simulink model "sensorless_pll_learning"  (R2025b)
settings: Solver=FixedStepDiscrete  StartTime=0.0  StopTime=1.99995  FixedStep=50e-6  RelTol=1e-3
InitFcn:
  | pll_prepare_demo_input
settings Model: Creator=16004  LastModifiedBy=16004

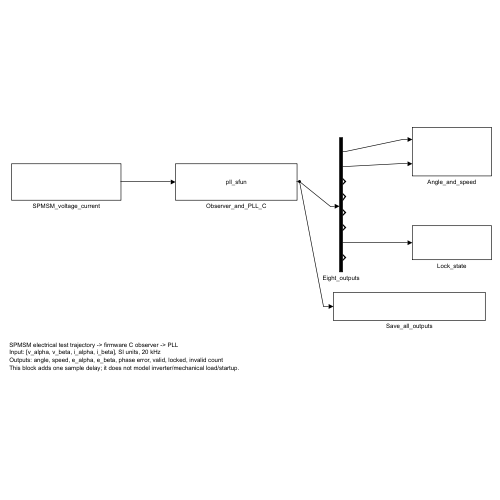
[thumbnail: Simulink's stored preview of the top-level diagram]
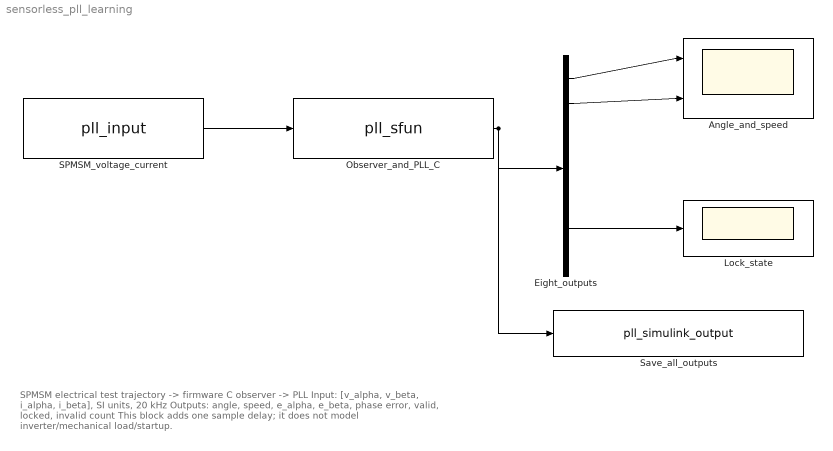
== system sensorless_pll_learning ==
  note: SPMSM electrical test trajectory -> firmware C observer -> PLL
      | Input: [v_alpha, v_beta, i_alpha, i_beta], SI units, 20 kHz
      | Outputs: angle, speed, e_alpha, e_beta, phase error, valid, locked, invalid count
      | This block adds one sample delay; it does not model inverter/mechanical load/startup.
  Angle_and_speed : Scope  NumInputPorts=2
  Eight_outputs : Demux  Outputs=8
  Lock_state : Scope
  Observer_and_PLL_C : M-S-Function  FunctionName=pll_sfun  Parameters=1
  SPMSM_voltage_current : FromWorkspace  VariableName=pll_input  Interpolate=off  OutputAfterFinalValue=Holding final value
  Save_all_outputs : ToWorkspace  VariableName=pll_simulink_output  SampleTime=-1
  wires:
  SPMSM_voltage_current/1 -> Observer_and_PLL_C/1
  Observer_and_PLL_C/1 -> Eight_outputs/1, Save_all_outputs/1
  Eight_outputs/1 -> Angle_and_speed/1
  Eight_outputs/2 -> Angle_and_speed/2
  Eight_outputs/7 -> Lock_state/1
